simulink model "modelLQR_histereza"  (R2015a)
settings: Solver=ode4  StartTime=0.0  StopTime=400  FixedStep=0.01  RelTol=1e-3
values from neighbouring files (symbols this model uses):
  h0 = 20    [NastawyLQR.m]    (also in SzukanieNastaw.m; wskaznikJakosci.m)
  K = lqr(A,B,Q,R)    [NastawyLQR.m]
  pompaP1 = p1    [SzukanieNastaw.m]
  ref = 20    [wskaznikJakosci.m]
  zaworP1 = [-49.1428571429 99.1142857143 -23.37]    [parametryWielomianuPWMZaworu.mat]
undefined symbols (not defined in the file or in its folder): sigbuilder_block, zaworC1, zaworC2
settings Model: Creator=konra  LastModifiedBy=konra

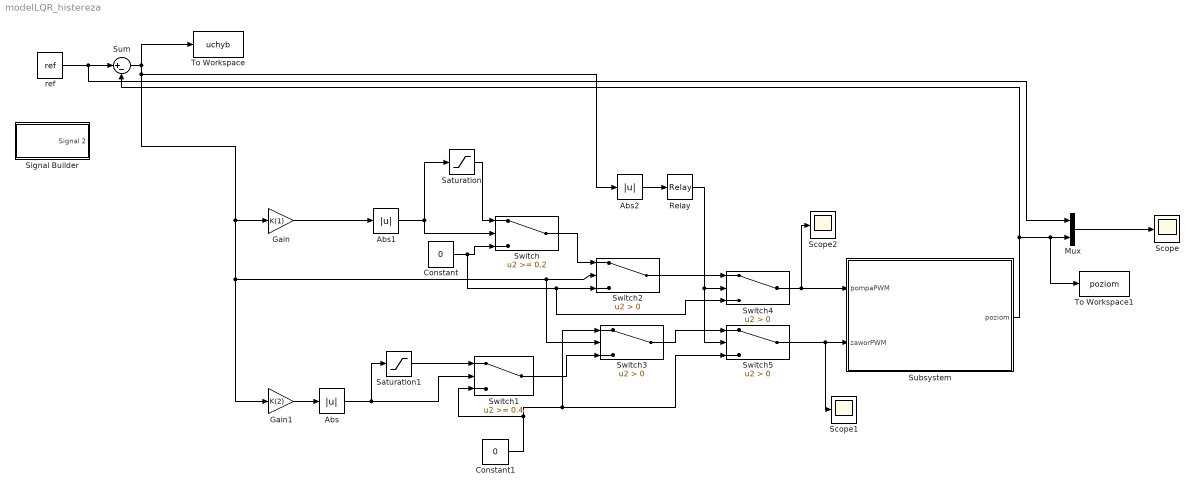
== system modelLQR_histereza ==
  Abs : Abs
  Abs1 : Abs
  Abs2 : Abs
  Constant : Constant  Value=0
  Constant1 : Constant  Value=0
  Gain : Gain  Gain=K(1)
  Gain1 : Gain  Gain=K(2)
  Mux : Mux  Inputs=2
  Relay : Relay  OnSwitchValue=3  OffSwitchValue=0
  Saturation : Saturate  UpperLimit=1  LowerLimit=0.2
  Saturation1 : Saturate  UpperLimit=1  LowerLimit=0.4
  Scope : Scope
  Scope1 : Scope
      settings: TimeRange=300  YMin=0  YMax=1  SaveName=ScopeData3
  Scope2 : Scope
      settings: SaveName=ScopeData4
  Signal Builder : Subsystem  Tag=STV Subsys  LoadFcn=sigbuilder_block('load');  StartFcn=sigbuilder_block('start');  StopFcn=sigbuilder_block('stop');  ClipboardFcn=sigbuilder_block('clipboard');  mask(Sigbuilder block){}
      mask help: Simulink:masks:SigbuilderBlock_MD
      mask init:
      | if ~strcmp(get_param(bdroot(gcbh),'SimulationStatus'),'stopped') tuvar = sigbuilder_block('maskInit'); end
      settings: CopyFcn=sigbuilder_block('copy');  DeleteFcn=sigbuilder_block('delete');  ModelCloseFcn=sigbuilder_block('modelClose');  PreSaveFcn=sigbuilder_block('preSave');  PauseFcn=sigbuilder_block('pause');  ContinueFcn=sigbuilder_block('continue');  NameChangeFcn=sigbuilder_block('namechange');  OpenFcn=sigbuilder_block('open',[437.6 199.2 550.4 400 ]);  CloseFcn=sigbuilder_block('close');
      mask Display: plot(0, 0, 100, 100,[2, 2, 32, 32, 2], [68, 8, 8, 68, 68],[32, 2], [38, 38], [32, 19, 2],[53, 60, 44], [32, 17, 17, 2],[16, 16, 31, 31]);txt = getActiveGroup(gcbh);text(2, 100, txt,'verticalAlignment', 'top');
  Subsystem : Subsystem
  Sum : Sum  Inputs=|+-
  Switch : Switch  Threshold=0.2
  Switch1 : Switch  Threshold=0.4
  Switch{2..5} (4 alike) : Switch  Criteria=u2 > Threshold
  To Workspace : ToWorkspace  VariableName=uchyb  SaveFormat=Structure With Time  SampleTime=-1
  To Workspace1 : ToWorkspace  VariableName=poziom  SaveFormat=Structure With Time  SampleTime=-1
  ref : Constant  Value=ref
  wires:
  Subsystem/1(poziom) -> To Workspace1/1, Mux/2, Sum/2
  Sum/1 -> Abs2/1, Gain/1, Gain1/1, Switch3/2, Switch2/2, To Workspace/1
  Saturation1/1 -> Switch1/1
  Saturation/1 -> Switch/1
  Switch/1 -> Switch2/1
  Switch1/1 -> Switch3/3
  Constant1/1 -> Switch3/1, Switch5/3, Switch1/3
  Gain1/1 -> Abs/1
  Switch2/1 -> Switch4/1
  Switch3/1 -> Switch5/1
  Gain/1 -> Abs1/1
  Abs1/1 -> Saturation/1, Switch/2
  Mux/1 -> Scope/1
  ref/1 -> Mux/1, Sum/1
  Switch4/1 -> Scope2/1, Subsystem/1(pompaPWM)
  Abs2/1 -> Relay/1
  Relay/1 -> Switch5/2, Switch4/2
  Switch5/1 -> Scope1/1, Subsystem/2(zaworPWM)
  Abs/1 -> Saturation1/1, Switch1/2
  Constant/1 -> Switch4/3, Switch2/3, Switch/3

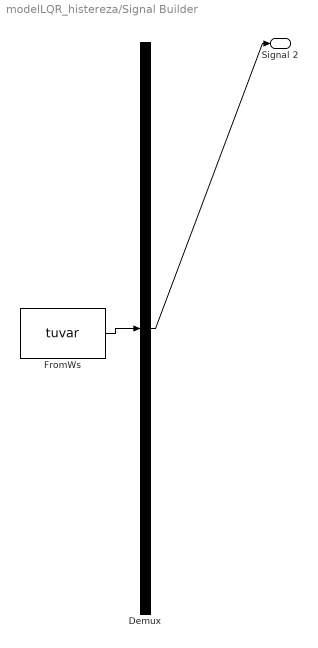
== system modelLQR_histereza/Signal Builder ==
  Demux : Demux  Tag=STV Demux  Outputs=1
  FromWs : FromWorkspace  Tag=STV FromWs  VariableName=tuvar  SampleTime=0
      SigBuilderData=|
      | common.afterFinalStr = 'Extrapolate'
      | common.sampleTime = 0
      | dataSet.timeRange = [0 300]
      | dataSet.name = 'Group 1'
      | sbobj.Groups.Name = 'Group 1'
      | sbobj.Groups.Signals.Name = 'Signal 2'
      | sbobj.Groups.Signals.XData = [0 80 80 300]
      | sbobj.Groups.Signals.YData = [30 30 5 5]
      | sbobj.Groups.TimeRange = [0 300]
  Signal 2 : Outport  Tag=STV Outport
  wires:
  FromWs/1 -> Demux/1
  Demux/1 -> Signal 2/1

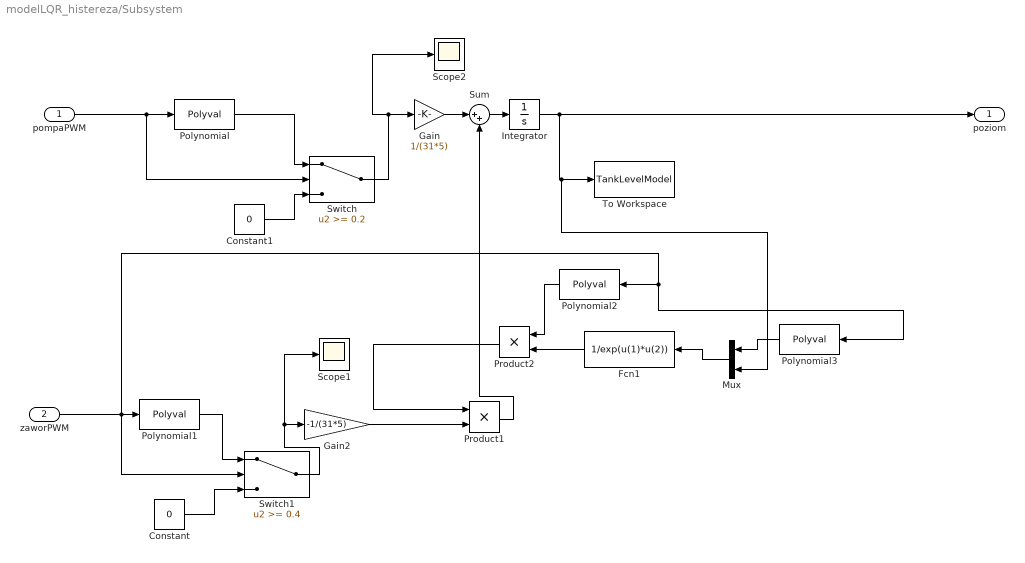
== system modelLQR_histereza/Subsystem ==
  pompaPWM : Inport
  zaworPWM : Inport  Port=2
  Constant : Constant  Value=0
  Constant1 : Constant  Value=0
  Fcn1 : Fcn  Expr=1/exp(u(1)*u(2))
  Gain : Gain  Gain=1/(31*5)
  Gain2 : Gain  Gain=-1/(31*5)
  Integrator : Integrator  InitialCondition=h0
  Mux : Mux  Inputs=2
  Polynomial : Polyval  Coefs=pompaP1
  Polynomial1 : Polyval  Coefs=zaworP1
  Polynomial2 : Polyval  Coefs=zaworC2
  Polynomial3 : Polyval  Coefs=zaworC1
  Product1 : Product
  Product2 : Product
  Scope1 : Scope
  Scope2 : Scope
      settings: SaveName=ScopeData2
  Sum : Sum  Inputs=|++
  Switch : Switch  Threshold=0.2
  Switch1 : Switch  Threshold=0.4
  To Workspace : ToWorkspace  VariableName=TankLevelModel  SaveFormat=Structure With Time  SampleTime=-1
  poziom : Outport
  wires:
  Switch1/1 -> Scope1/1, Gain2/1
  Polynomial1/1 -> Switch1/1
  Constant/1 -> Switch1/3
  Polynomial/1 -> Switch/1
  Constant1/1 -> Switch/3
  Switch/1 -> Scope2/1, Gain/1
  pompaPWM/1 -> Switch/2, Polynomial/1
  Gain2/1 -> Product1/2
  Product1/1 -> Sum/2
  Product2/1 -> Product1/1
  Integrator/1 -> poziom/1, Mux/2, To Workspace/1
  Fcn1/1 -> Product2/2
  zaworPWM/1 -> Switch1/2, Polynomial1/1, Polynomial3/1, Polynomial2/1
  Polynomial2/1 -> Product2/1
  Mux/1 -> Fcn1/1
  Polynomial3/1 -> Mux/1
  Gain/1 -> Sum/1
  Sum/1 -> Integrator/1
